simulink model "Simulator_nonlinear_inversion"  (R2015a)
settings: Solver=ode45  StartTime=0.0  StopTime=10  RelTol=1e-3
values from neighbouring files (symbols this model uses):
  A_Servo = [0 1 0; 0 0 1 ; -B0/B3 -B1/B3 -B2/B3]    [Parameters.m]
  b = 0.55/2    (= 0.275)    [Parameters.m]
  B_Servo = [0 ; 0 ; B0/B3]    [Parameters.m]
  C_Servo = eye(3)    [Parameters.m]
  dLMN = [dLdp  0    0 ... (first row only)    [Parameters.m]
  g = 9.81    [Parameters.m]
  I_Pi = diag([8.450e-5 8.450e-5 4.580e-5])    [Parameters.m]
  In = diag([Ixx Iyy Izz])    [Parameters.m]
  InInv = In\eye(3)    [Parameters.m]
  KaD = 5.4    [Parameters.m]
  KaI = 3.6    [Parameters.m]
  KaN = 38    [Parameters.m]
  KaP = 8.0    (= 8)    [Parameters.m]
  Kba = sqrt(KaD/KaI)    [Parameters.m]
  Kbp = sqrt(Kdp/Kip)    [Parameters.m]
  Kbq = sqrt(Kdq/Kiq)    [Parameters.m]
  Kbr = sqrt(Kdr/Kir)    [Parameters.m]
  Kdp = 0.0499    [Parameters.m]
  Kdq = 0.0499    [Parameters.m]
  Kdr = 0.0153    [Parameters.m]
  Kip = 0.304    [Parameters.m]
  Kiq = 0.304    [Parameters.m]
  Kir = 0.125    [Parameters.m]
  KPD = 0.00512    [Parameters.m]
  KPP = 1.61    [Parameters.m]
  Kpp = 0.298    [Parameters.m]
  Kpq = 0.298    [Parameters.m]
  Kpr = 0.135    [Parameters.m]
  Kq = Cq*ro*A*R^3    (= 2.88925724261e-07)    [Parameters.m]
  KRD = 0.00512    [Parameters.m]
  KRP = 1.61    [Parameters.m]
  Kt = Ct*ro*A*R^2    (= 2.46191978476e-05)    [Parameters.m]
  m = 1.510    (= 1.51)    [Parameters.m]
  m_servo = p(1)    [Parameters.m]    (also in model_test_signals.m = 572.9578)
  Mb = diag([m m m])    [Parameters.m]
  MbInv = Mb\eye(3)    [Parameters.m]
  N = 1/Tf    (= 100)    [Parameters.m]
  omega_hover = OMEhov    [Parameters.m]
  pitchMax = pi/6    (= 0.523598775598)    [Parameters.m]
  q_servo = p(2)    [Parameters.m]    (also in model_test_signals.m = 1500)
  rollMax = pi/6    (= 0.523598775598)    [Parameters.m]
  satp = 1.5    [Parameters.m]
  satq = 1.5    [Parameters.m]
  satr = 1    [Parameters.m]
  tau = 0.055257    [Parameters.m]
  U = [-1; 0; 0; 0]    [Main.m]
  x1 = [m q]    [Parameters.m]
  yawRateMax = pi/2    (= 1.57079632679)    [Parameters.m]
undefined symbols (not defined in the file or in its folder): KPI, KRI, sigbuilder_block
libraries: simulink x10, aerolibutil x10
(part 2 of 3)

== system Simulator_nonlinear_inversion/TiltCopter/Actuators/External Momentum_2 ==
  tau_pi : Inport
  alpha_i : Inport  Port=2
  omega_i : Inport  Port=3
  motor_number : Inport  Port=4
  3x3 Cross Product : aerolibutil/3x3 Cross Product
  O_BPi : MATLAB Function  TreatAsAtomicUnit=on
  Product : Product  Multiplication=Matrix(*)
  Product1 : Product  Multiplication=Matrix(*)
  R_BP2 : MATLAB Function  TreatAsAtomicUnit=on
  Sum : Sum  Inputs=-+|
  Thrust computation : Subsystem
  M_i : Outport
  wires:
  Sum/1 -> M_i/1
  R_BP2/1(Rotation_matrix) -> Product1/1, Product/1
  alpha_i/1 -> R_BP2/1(alpha_2)
  Product/1 -> 3x3 Cross Product/2
  tau_pi/1 -> Product1/2
  motor_number/1 -> O_BPi/1(motor_number)
  omega_i/1 -> Thrust computation/1(omega_i)
  Thrust computation/1(Vector_Thrust_i) -> Product/2
  3x3 Cross Product/1 -> Sum/2
  Product1/1 -> Sum/1
  O_BPi/1(Origin_Rotation) -> 3x3 Cross Product/1

== system Simulator_nonlinear_inversion/TiltCopter/Actuators/External Momentum_3 ==
  tau_pi : Inport
  alpha_i : Inport  Port=2
  omega_i : Inport  Port=3
  motor_number : Inport  Port=4
  3x3 Cross Product : aerolibutil/3x3 Cross Product
  O_BPi : MATLAB Function  TreatAsAtomicUnit=on
  Product : Product  Multiplication=Matrix(*)
  Product1 : Product  Multiplication=Matrix(*)
  R_BP3 : MATLAB Function  TreatAsAtomicUnit=on
  Sum : Sum  Inputs=-+|
  Thrust computation : Subsystem
  M_i : Outport
  wires:
  Sum/1 -> M_i/1
  R_BP3/1(Rotation_matrix) -> Product1/1, Product/1
  alpha_i/1 -> R_BP3/1(alpha_3)
  Product/1 -> 3x3 Cross Product/2
  tau_pi/1 -> Product1/2
  motor_number/1 -> O_BPi/1(motor_number)
  omega_i/1 -> Thrust computation/1(omega_i)
  Thrust computation/1(Vector_Thrust_i) -> Product/2
  3x3 Cross Product/1 -> Sum/2
  Product1/1 -> Sum/1
  O_BPi/1(Origin_Rotation) -> 3x3 Cross Product/1

== system Simulator_nonlinear_inversion/TiltCopter/Actuators/External Momentum_4 ==
  tau_pi : Inport
  alpha_i : Inport  Port=2
  omega_i : Inport  Port=3
  motor_number : Inport  Port=4
  3x3 Cross Product : aerolibutil/3x3 Cross Product
  O_BPi : MATLAB Function  TreatAsAtomicUnit=on
  Product : Product  Multiplication=Matrix(*)
  Product1 : Product  Multiplication=Matrix(*)
  R_BP4 : MATLAB Function  TreatAsAtomicUnit=on
  Sum : Sum  Inputs=-+|
  Thrust computation : Subsystem
  M_i : Outport
  wires:
  Sum/1 -> M_i/1
  R_BP4/1(Rotation_matrix) -> Product1/1, Product/1
  alpha_i/1 -> R_BP4/1(alpha_4)
  Product/1 -> 3x3 Cross Product/2
  tau_pi/1 -> Product1/2
  motor_number/1 -> O_BPi/1(motor_number)
  omega_i/1 -> Thrust computation/1(omega_i)
  Thrust computation/1(Vector_Thrust_i) -> Product/2
  3x3 Cross Product/1 -> Sum/2
  Product1/1 -> Sum/1
  O_BPi/1(Origin_Rotation) -> 3x3 Cross Product/1

== system Simulator_nonlinear_inversion/TiltCopter/Actuators/Servo_Motor 1 ==
  Alpha_1 [deg] : Inport
  Demux : Demux  Outputs=3
  State-Space : StateSpace  A=A_Servo  B=B_Servo  C=C_Servo  D=[0 0 0]'  X0=[0 0 0 ]  ContinuousStateAttributes=['alpha' 'dalpha' 'ddalpha']
  deg2rad : Gain  Gain=pi/180
  alpha_1 [rad] : Outport
  dalpha_1 : Outport  Port=2
  ddalpha_1 : Outport  Port=3
  wires:
  deg2rad/1 -> State-Space/1
  Alpha_1 [deg]/1 -> deg2rad/1
  State-Space/1 -> Demux/1
  Demux/1 -> alpha_1 [rad]/1
  Demux/2 -> dalpha_1/1
  Demux/3 -> ddalpha_1/1

== system Simulator_nonlinear_inversion/TiltCopter/Actuators/Servo_Motor 2 ==
  Alpha_2 [deg] : Inport
  Demux : Demux  Outputs=3
  State-Space : StateSpace  A=A_Servo  B=B_Servo  C=C_Servo  D=[0 0 0]'  X0=[0 0 0 ]  ContinuousStateAttributes=['alpha' 'dalpha' 'ddalpha']
  deg2rad : Gain  Gain=pi/180
  alpha_2 [rad] : Outport
  dalpha_2 : Outport  Port=2
  ddalpha_2 : Outport  Port=3
  wires:
  State-Space/1 -> Demux/1
  Demux/3 -> ddalpha_2/1
  Demux/2 -> dalpha_2/1
  Demux/1 -> alpha_2 [rad]/1
  deg2rad/1 -> State-Space/1
  Alpha_2 [deg]/1 -> deg2rad/1

== system Simulator_nonlinear_inversion/TiltCopter/Actuators/Servo_Motor 3 ==
  Alpha_3 [deg] : Inport
  Demux : Demux  Outputs=3
  State-Space : StateSpace  A=A_Servo  B=B_Servo  C=C_Servo  D=[0 0 0]'  X0=[0 0 0 ]  ContinuousStateAttributes=['alpha' 'dalpha' 'ddalpha']
  deg2rad : Gain  Gain=pi/180
  alpha_3 [rad] : Outport
  dalpha_3 : Outport  Port=2
  ddalpha_3 : Outport  Port=3
  wires:
  Demux/1 -> alpha_3 [rad]/1
  Demux/2 -> dalpha_3/1
  Demux/3 -> ddalpha_3/1
  deg2rad/1 -> State-Space/1
  Alpha_3 [deg]/1 -> deg2rad/1
  State-Space/1 -> Demux/1

== system Simulator_nonlinear_inversion/TiltCopter/Actuators/Servo_Motor 4 ==
  Alpha_4 [deg] : Inport
  Demux : Demux  Outputs=3
  State-Space : StateSpace  A=A_Servo  B=B_Servo  C=C_Servo  D=[0 0 0]'  X0=[0 0 0 ]  ContinuousStateAttributes=['alpha' 'dalpha' 'ddalpha']
  deg2rad : Gain  Gain=pi/180
  alpha_4 [rad] : Outport
  dalpha_4 : Outport  Port=2
  ddalpha_4 : Outport  Port=3
  wires:
  Demux/1 -> alpha_4 [rad]/1
  Demux/2 -> dalpha_4/1
  Demux/3 -> ddalpha_4/1
  deg2rad/1 -> State-Space/1
  Alpha_4 [deg]/1 -> deg2rad/1
  State-Space/1 -> Demux/1

== system Simulator_nonlinear_inversion/TiltCopter/Actuators/Traslational Force_1 ==
  alpha_i : Inport
  omega_i : Inport  Port=2
  Product : Product  Multiplication=Matrix(*)
  R_BP1 : MATLAB Function  TreatAsAtomicUnit=on
  Thrust computation : Subsystem
  F_i : Outport
  wires:
  Thrust computation/1(Vector_Thrust_i) -> Product/2
  Product/1 -> F_i/1
  omega_i/1 -> Thrust computation/1(omega_i)
  R_BP1/1(Rotation_matrix) -> Product/1
  alpha_i/1 -> R_BP1/1(alpha_1)

== system Simulator_nonlinear_inversion/TiltCopter/Actuators/Traslational Force_2 ==
  alpha_i : Inport
  omega_i : Inport  Port=2
  Product : Product  Multiplication=Matrix(*)
  R_BP2 : MATLAB Function  TreatAsAtomicUnit=on
  Thrust computation : Subsystem
  F_i : Outport
  wires:
  Thrust computation/1(Vector_Thrust_i) -> Product/2
  Product/1 -> F_i/1
  omega_i/1 -> Thrust computation/1(omega_i)
  R_BP2/1(Rotation_matrix) -> Product/1
  alpha_i/1 -> R_BP2/1(alpha_2)

== system Simulator_nonlinear_inversion/TiltCopter/Actuators/Traslational Force_3 ==
  alpha_i : Inport
  omega_i : Inport  Port=2
  Product : Product  Multiplication=Matrix(*)
  R_BP3 : MATLAB Function  TreatAsAtomicUnit=on
  Thrust computation : Subsystem
  F_i : Outport
  wires:
  Thrust computation/1(Vector_Thrust_i) -> Product/2
  Product/1 -> F_i/1
  omega_i/1 -> Thrust computation/1(omega_i)
  R_BP3/1(Rotation_matrix) -> Product/1
  alpha_i/1 -> R_BP3/1(alpha_3)

== system Simulator_nonlinear_inversion/TiltCopter/Actuators/Traslational Force_4 ==
  alpha_i : Inport
  omega_i : Inport  Port=2
  Product : Product  Multiplication=Matrix(*)
  R_BP4 : MATLAB Function  TreatAsAtomicUnit=on
  Thrust computation : Subsystem
  F_i : Outport
  wires:
  Thrust computation/1(Vector_Thrust_i) -> Product/2
  Product/1 -> F_i/1
  omega_i/1 -> Thrust computation/1(omega_i)
  R_BP4/1(Rotation_matrix) -> Product/1
  alpha_i/1 -> R_BP4/1(alpha_4)

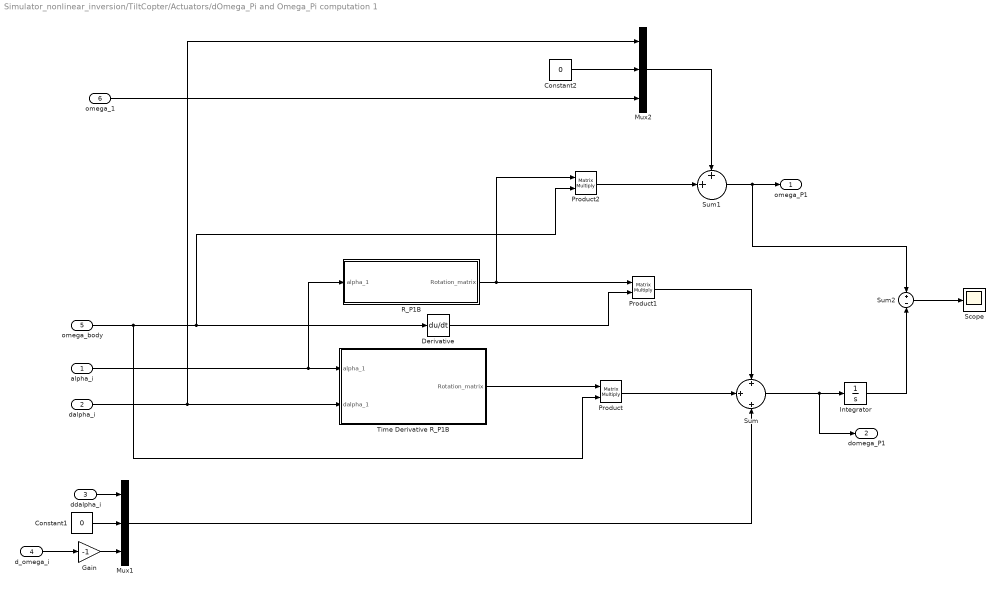
== system Simulator_nonlinear_inversion/TiltCopter/Actuators/dOmega_Pi and Omega_Pi computation 1 ==
  alpha_i : Inport
  dalpha_i : Inport  Port=2
  ddalpha_i : Inport  Port=3
  d_omega_i : Inport  Port=4
  omega_body : Inport  Port=5
  omega_1 : Inport  Port=6
  Constant1 : Constant  Value=0
  Constant2 : Constant  Value=0
  Derivative : Derivative
  Gain : Gain  Gain=-1
  Integrator : Integrator
  Mux1 : Mux  Inputs=3
  Mux2 : Mux  Inputs=3
  Product : Product  Multiplication=Matrix(*)
  Product1 : Product  Multiplication=Matrix(*)
  Product2 : Product  Multiplication=Matrix(*)
  R_P1B : MATLAB Function  TreatAsAtomicUnit=on
  Scope : Scope
      settings: ShowLegends=on  YMin=-10  YMax=10  SaveName=ScopeData29
  Sum : Sum  Inputs=+|+|+
  Sum1 : Sum  Inputs=++|
  Sum2 : Sum  Inputs=+-
  Time Derivative R_P1B : MATLAB Function  TreatAsAtomicUnit=on
  omega_P1 : Outport
  domega_P1 : Outport  Port=2
  wires:
  Derivative/1 -> Product1/2
  Product/1 -> Sum/2
  Time Derivative R_P1B/1(Rotation_matrix) -> Product/1
  Constant1/1 -> Mux1/2
  omega_body/1 -> Product/2, Product2/2, Derivative/1
  dalpha_i/1 -> Mux2/1, Time Derivative R_P1B/2(dalpha_1)
  alpha_i/1 -> R_P1B/1(alpha_1), Time Derivative R_P1B/1(alpha_1)
  R_P1B/1(Rotation_matrix) -> Product2/1, Product1/1
  Sum/1 -> domega_P1/1, Integrator/1
  Product1/1 -> Sum/1
  Mux1/1 -> Sum/3
  ddalpha_i/1 -> Mux1/1
  Product2/1 -> Sum1/2
  Constant2/1 -> Mux2/2
  Mux2/1 -> Sum1/1
  Sum1/1 -> Sum2/1, omega_P1/1
  omega_1/1 -> Mux2/3
  d_omega_i/1 -> Gain/1
  Integrator/1 -> Sum2/2
  Sum2/1 -> Scope/1
  Gain/1 -> Mux1/3

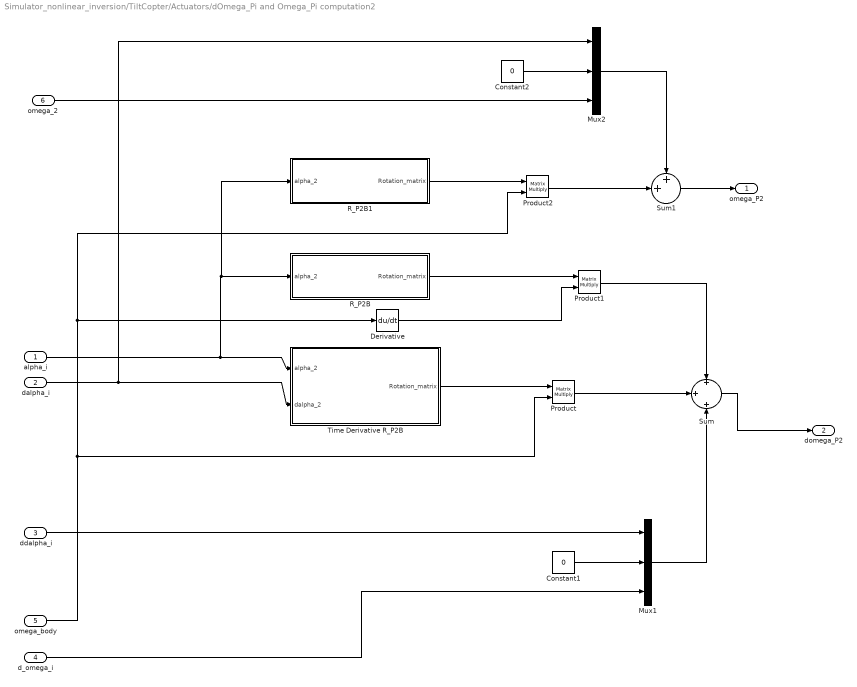
== system Simulator_nonlinear_inversion/TiltCopter/Actuators/dOmega_Pi and Omega_Pi computation2 ==
  alpha_i : Inport
  dalpha_i : Inport  Port=2
  ddalpha_i : Inport  Port=3
  d_omega_i : Inport  Port=4
  omega_body : Inport  Port=5
  omega_2 : Inport  Port=6
  Constant1 : Constant  Value=0
  Constant2 : Constant  Value=0
  Derivative : Derivative
  Mux1 : Mux  Inputs=3
  Mux2 : Mux  Inputs=3
  Product : Product  Multiplication=Matrix(*)
  Product1 : Product  Multiplication=Matrix(*)
  Product2 : Product  Multiplication=Matrix(*)
  R_P2B : MATLAB Function  TreatAsAtomicUnit=on
  R_P2B1 : MATLAB Function  TreatAsAtomicUnit=on
  Sum : Sum  Inputs=+|+|+
  Sum1 : Sum  Inputs=++|
  Time Derivative R_P2B : MATLAB Function  TreatAsAtomicUnit=on
  omega_P2 : Outport
  domega_P2 : Outport  Port=2
  wires:
  Derivative/1 -> Product1/2
  Product/1 -> Sum/2
  Time Derivative R_P2B/1(Rotation_matrix) -> Product/1
  Constant1/1 -> Mux1/2
  omega_body/1 -> Product/2, Product2/2, Derivative/1
  dalpha_i/1 -> Mux2/1, Time Derivative R_P2B/2(dalpha_2)
  alpha_i/1 -> R_P2B1/1(alpha_2), R_P2B/1(alpha_2), Time Derivative R_P2B/1(alpha_2)
  Sum/1 -> domega_P2/1
  Product1/1 -> Sum/1
  Mux1/1 -> Sum/3
  ddalpha_i/1 -> Mux1/1
  R_P2B/1(Rotation_matrix) -> Product1/1
  R_P2B1/1(Rotation_matrix) -> Product2/1
  Product2/1 -> Sum1/2
  Constant2/1 -> Mux2/2
  Mux2/1 -> Sum1/1
  Sum1/1 -> omega_P2/1
  d_omega_i/1 -> Mux1/3
  omega_2/1 -> Mux2/3

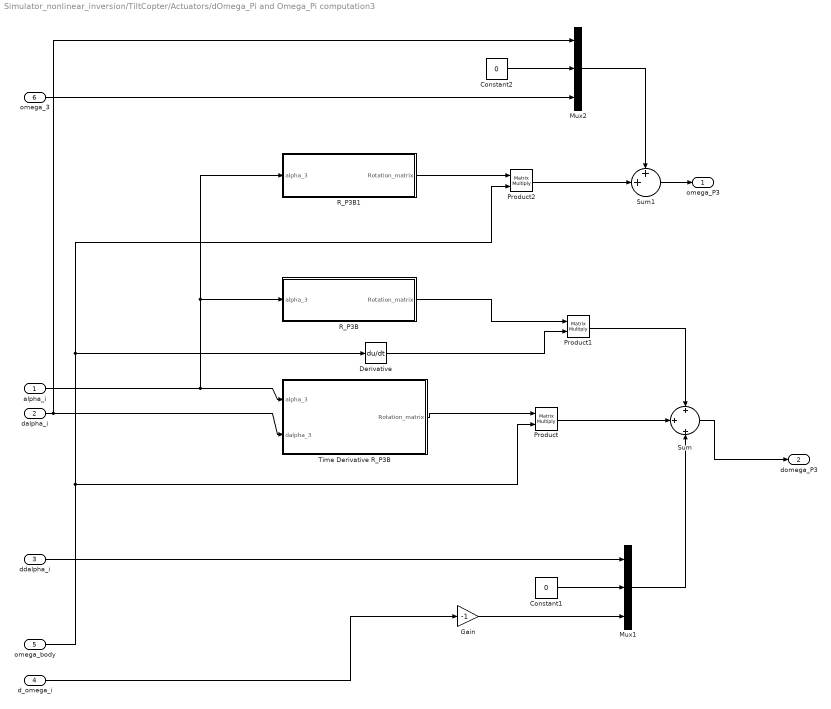
== system Simulator_nonlinear_inversion/TiltCopter/Actuators/dOmega_Pi and Omega_Pi computation3 ==
  alpha_i : Inport
  dalpha_i : Inport  Port=2
  ddalpha_i : Inport  Port=3
  d_omega_i : Inport  Port=4
  omega_body : Inport  Port=5
  omega_3 : Inport  Port=6
  Constant1 : Constant  Value=0
  Constant2 : Constant  Value=0
  Derivative : Derivative
  Gain : Gain  Gain=-1
  Mux1 : Mux  Inputs=3
  Mux2 : Mux  Inputs=3
  Product : Product  Multiplication=Matrix(*)
  Product1 : Product  Multiplication=Matrix(*)
  Product2 : Product  Multiplication=Matrix(*)
  R_P3B : MATLAB Function  TreatAsAtomicUnit=on
  R_P3B1 : MATLAB Function  TreatAsAtomicUnit=on
  Sum : Sum  Inputs=+|+|+
  Sum1 : Sum  Inputs=++|
  Time Derivative R_P3B : MATLAB Function  TreatAsAtomicUnit=on
  omega_P3 : Outport
  domega_P3 : Outport  Port=2
  wires:
  Derivative/1 -> Product1/2
  Product/1 -> Sum/2
  Time Derivative R_P3B/1(Rotation_matrix) -> Product/1
  Constant1/1 -> Mux1/2
  omega_body/1 -> Product/2, Product2/2, Derivative/1
  alpha_i/1 -> R_P3B1/1(alpha_3), R_P3B/1(alpha_3), Time Derivative R_P3B/1(alpha_3)
  Sum/1 -> domega_P3/1
  Product1/1 -> Sum/1
  Mux1/1 -> Sum/3
  ddalpha_i/1 -> Mux1/1
  R_P3B/1(Rotation_matrix) -> Product1/1
  R_P3B1/1(Rotation_matrix) -> Product2/1
  Product2/1 -> Sum1/2
  Constant2/1 -> Mux2/2
  Mux2/1 -> Sum1/1
  dalpha_i/1 -> Mux2/1, Time Derivative R_P3B/2(dalpha_3)
  Sum1/1 -> omega_P3/1
  d_omega_i/1 -> Gain/1
  omega_3/1 -> Mux2/3
  Gain/1 -> Mux1/3

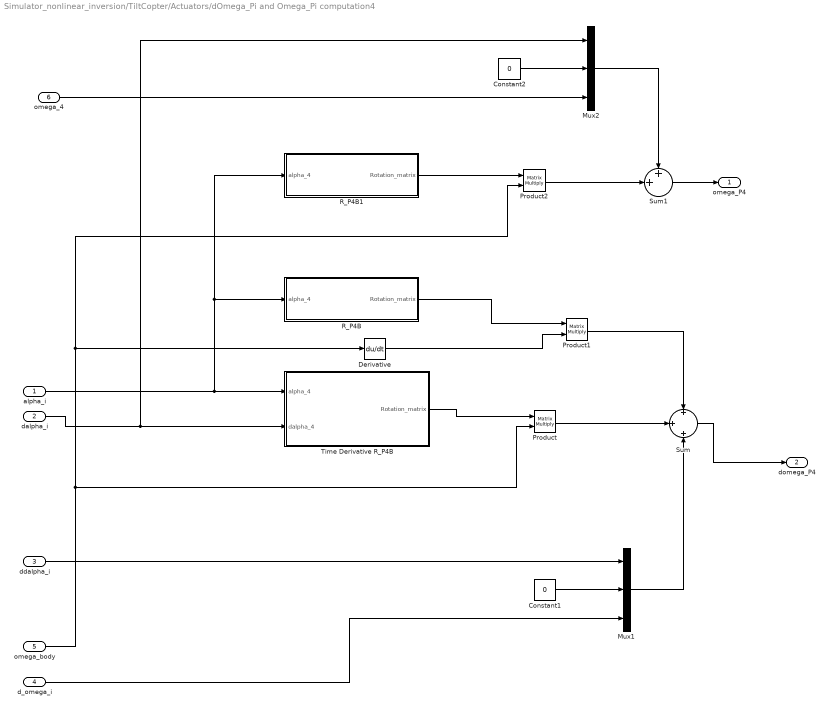
== system Simulator_nonlinear_inversion/TiltCopter/Actuators/dOmega_Pi and Omega_Pi computation4 ==
  alpha_i : Inport
  dalpha_i : Inport  Port=2
  ddalpha_i : Inport  Port=3
  d_omega_i : Inport  Port=4
  omega_body : Inport  Port=5
  omega_4 : Inport  Port=6
  Constant1 : Constant  Value=0
  Constant2 : Constant  Value=0
  Derivative : Derivative
  Mux1 : Mux  Inputs=3
  Mux2 : Mux  Inputs=3
  Product : Product  Multiplication=Matrix(*)
  Product1 : Product  Multiplication=Matrix(*)
  Product2 : Product  Multiplication=Matrix(*)
  R_P4B : MATLAB Function  TreatAsAtomicUnit=on
  R_P4B1 : MATLAB Function  TreatAsAtomicUnit=on
  Sum : Sum  Inputs=+|+|+
  Sum1 : Sum  Inputs=++|
  Time Derivative R_P4B : MATLAB Function  TreatAsAtomicUnit=on
  omega_P4 : Outport
  domega_P4 : Outport  Port=2
  wires:
  Derivative/1 -> Product1/2
  Product/1 -> Sum/2
  Time Derivative R_P4B/1(Rotation_matrix) -> Product/1
  Constant1/1 -> Mux1/2
  omega_body/1 -> Product/2, Product2/2, Derivative/1
  dalpha_i/1 -> Mux2/1, Time Derivative R_P4B/2(dalpha_4)
  alpha_i/1 -> R_P4B1/1(alpha_4), R_P4B/1(alpha_4), Time Derivative R_P4B/1(alpha_4)
  Sum/1 -> domega_P4/1
  Product1/1 -> Sum/1
  Mux1/1 -> Sum/3
  ddalpha_i/1 -> Mux1/1
  R_P4B/1(Rotation_matrix) -> Product1/1
  Product2/1 -> Sum1/2
  Constant2/1 -> Mux2/2
  Mux2/1 -> Sum1/1
  R_P4B1/1(Rotation_matrix) -> Product2/1
  Sum1/1 -> omega_P4/1
  omega_4/1 -> Mux2/3
  d_omega_i/1 -> Mux1/3

== system Simulator_nonlinear_inversion/TiltCopter/Actuators/tau_p1 computation ==
  omega_P1 : Inport
  domega_P1 : Inport  Port=2
  omega_i : Inport  Port=3
  3x3 Cross Product : aerolibutil/3x3 Cross Product
  Constant : Constant  Value=I_Pi
  Drag torque computation : Subsystem
  Gain : Gain  Gain=[1;1;-1]
  Product : Product  Multiplication=Matrix(*)
  Product1 : Product  Multiplication=Matrix(*)
  Sum : Sum  Inputs=+|+|-
  tau_P1 : Outport
  wires:
  Constant/1 -> Product/1, Product1/1
  omega_P1/1 -> 3x3 Cross Product/1, Product1/2
  Product/1 -> Sum/2
  domega_P1/1 -> Product/2
  Product1/1 -> 3x3 Cross Product/2
  Sum/1 -> tau_P1/1
  3x3 Cross Product/1 -> Sum/1
  Drag torque computation/1(Vector_DragTorque_i) -> Gain/1
  omega_i/1 -> Drag torque computation/1(omega_P1_z)
  Gain/1 -> Sum/3

== system Simulator_nonlinear_inversion/TiltCopter/Actuators/tau_p2 computation ==
  omega_P2 : Inport
  domega_P2 : Inport  Port=2
  omega_i : Inport  Port=3
  3x3 Cross Product : aerolibutil/3x3 Cross Product
  Constant : Constant  Value=I_Pi
  Drag torque computation : Subsystem
  Gain : Gain  Gain=[1;1;-1]
  Product : Product  Multiplication=Matrix(*)
  Product1 : Product  Multiplication=Matrix(*)
  Sum : Sum  Inputs=+|+|-
  tau_P2 : Outport
  wires:
  3x3 Cross Product/1 -> Sum/1
  Sum/1 -> tau_P2/1
  Product1/1 -> 3x3 Cross Product/2
  domega_P2/1 -> Product/2
  Product/1 -> Sum/2
  omega_P2/1 -> Product1/2, 3x3 Cross Product/1
  Constant/1 -> Product/1, Product1/1
  Drag torque computation/1(Vector_DragTorque_i) -> Gain/1
  omega_i/1 -> Drag torque computation/1(omega_P2)
  Gain/1 -> Sum/3

== system Simulator_nonlinear_inversion/TiltCopter/Actuators/tau_p3 computation1 ==
  omega_P3 : Inport
  domega_P3 : Inport  Port=2
  omega_i : Inport  Port=3
  3x3 Cross Product : aerolibutil/3x3 Cross Product
  Constant : Constant  Value=I_Pi
  Drag torque computation : Subsystem
  Gain : Gain  Gain=[1;1;-1]
  Product : Product  Multiplication=Matrix(*)
  Product1 : Product  Multiplication=Matrix(*)
  Sum : Sum  Inputs=+|+|-
  tau_P3 : Outport
  wires:
  Constant/1 -> Product1/1, Product/1
  omega_P3/1 -> 3x3 Cross Product/1, Product1/2
  Product/1 -> Sum/2
  domega_P3/1 -> Product/2
  Product1/1 -> 3x3 Cross Product/2
  Sum/1 -> tau_P3/1
  3x3 Cross Product/1 -> Sum/1
  Drag torque computation/1(Vector_DragTorque_i) -> Gain/1
  omega_i/1 -> Drag torque computation/1(omega_P3)
  Gain/1 -> Sum/3

== system Simulator_nonlinear_inversion/TiltCopter/Actuators/tau_p4 computation2 ==
  omega_P4 : Inport
  domega_P4 : Inport  Port=2
  omega_i : Inport  Port=3
  3x3 Cross Product : aerolibutil/3x3 Cross Product
  Constant : Constant  Value=I_Pi
  Drag torque computation : Subsystem
  Gain : Gain  Gain=[1;1;-1]
  Product : Product  Multiplication=Matrix(*)
  Product1 : Product  Multiplication=Matrix(*)
  Sum : Sum  Inputs=+|+|-
  tau_P4 : Outport
  wires:
  3x3 Cross Product/1 -> Sum/1
  Sum/1 -> tau_P4/1
  Product1/1 -> 3x3 Cross Product/2
  domega_P4/1 -> Product/2
  Product/1 -> Sum/2
  omega_P4/1 -> Product1/2, 3x3 Cross Product/1
  Constant/1 -> Product/1, Product1/1
  Drag torque computation/1(Vector_DragTorque_i) -> Gain/1
  omega_i/1 -> Drag torque computation/1(omega_P4)
  Gain/1 -> Sum/3

== system Simulator_nonlinear_inversion/TiltCopter/Actuators/ESC+Brushless1/Subsystem ==
  Throttle [%] : Inport
  Bias : Bias  Bias=x1(2)
  Gain : Gain  Gain=x1(1)
  Gain1 : Gain  Gain=-1/tau
  Gain2 : Gain  Gain=1/tau
  Gain3 : Gain  Gain=x1(1)
  Gain4 : Gain  Gain=x1(1)
  Sum : Sum  Inputs=|++
  Transfer Fcn : TransferFcn  Denominator=[(tau) 1]
  Transfer Fcn1 : TransferFcn  Denominator=[(tau) 1]
  omega_i : Outport
  domega_i : Outport  Port=2
  wires:
  Throttle [%]/1 -> Gain4/1, Transfer Fcn1/1, Transfer Fcn/1
  Transfer Fcn1/1 -> Gain1/1
  Gain1/1 -> Gain3/1
  Sum/1 -> domega_i/1
  Gain2/1 -> Sum/2
  Gain3/1 -> Sum/1
  Bias/1 -> omega_i/1
  Gain/1 -> Bias/1
  Transfer Fcn/1 -> Gain/1
  Gain4/1 -> Gain2/1

== system Simulator_nonlinear_inversion/TiltCopter/Actuators/ESC+Brushless2/Subsystem ==
  Throttle [%] : Inport
  Bias : Bias  Bias=x1(2)
  Gain : Gain  Gain=x1(1)
  Gain1 : Gain  Gain=-1/tau
  Gain2 : Gain  Gain=1/tau
  Gain3 : Gain  Gain=x1(1)
  Gain4 : Gain  Gain=x1(1)
  Sum : Sum  Inputs=|++
  Transfer Fcn : TransferFcn  Denominator=[(tau) 1]
  Transfer Fcn1 : TransferFcn  Denominator=[(tau) 1]
  omega_i : Outport
  domega_i : Outport  Port=2
  wires:
  Throttle [%]/1 -> Gain4/1, Transfer Fcn1/1, Transfer Fcn/1
  Transfer Fcn1/1 -> Gain1/1
  Gain1/1 -> Gain3/1
  Sum/1 -> domega_i/1
  Gain2/1 -> Sum/2
  Gain3/1 -> Sum/1
  Bias/1 -> omega_i/1
  Gain/1 -> Bias/1
  Transfer Fcn/1 -> Gain/1
  Gain4/1 -> Gain2/1

== system Simulator_nonlinear_inversion/TiltCopter/Actuators/ESC+Brushless3/Subsystem ==
  Throttle [%] : Inport
  Bias : Bias  Bias=x1(2)
  Gain : Gain  Gain=x1(1)
  Gain1 : Gain  Gain=-1/tau
  Gain2 : Gain  Gain=1/tau
  Gain3 : Gain  Gain=x1(1)
  Gain4 : Gain  Gain=x1(1)
  Sum : Sum  Inputs=|++
  Transfer Fcn : TransferFcn  Denominator=[(tau) 1]
  Transfer Fcn1 : TransferFcn  Denominator=[(tau) 1]
  omega_i : Outport
  domega_i : Outport  Port=2
  wires:
  Throttle [%]/1 -> Gain4/1, Transfer Fcn1/1, Transfer Fcn/1
  Transfer Fcn1/1 -> Gain1/1
  Gain1/1 -> Gain3/1
  Sum/1 -> domega_i/1
  Gain2/1 -> Sum/2
  Gain3/1 -> Sum/1
  Bias/1 -> omega_i/1
  Gain/1 -> Bias/1
  Transfer Fcn/1 -> Gain/1
  Gain4/1 -> Gain2/1

== system Simulator_nonlinear_inversion/TiltCopter/Actuators/ESC+Brushless4/Subsystem ==
  Throttle [%] : Inport
  Bias : Bias  Bias=x1(2)
  Gain : Gain  Gain=x1(1)
  Gain1 : Gain  Gain=-1/tau
  Gain2 : Gain  Gain=1/tau
  Gain3 : Gain  Gain=x1(1)
  Gain4 : Gain  Gain=x1(1)
  Sum : Sum  Inputs=|++
  Transfer Fcn : TransferFcn  Denominator=[(tau) 1]
  Transfer Fcn1 : TransferFcn  Denominator=[(tau) 1]
  omega_i : Outport
  domega_i : Outport  Port=2
  wires:
  Throttle [%]/1 -> Gain4/1, Transfer Fcn1/1, Transfer Fcn/1
  Transfer Fcn1/1 -> Gain1/1
  Gain1/1 -> Gain3/1
  Sum/1 -> domega_i/1
  Gain2/1 -> Sum/2
  Gain3/1 -> Sum/1
  Bias/1 -> omega_i/1
  Gain/1 -> Bias/1
  Transfer Fcn/1 -> Gain/1
  Gain4/1 -> Gain2/1

== system Simulator_nonlinear_inversion/TiltCopter/Actuators/External Momentum_1/Thrust computation ==
  omega_i : Inport
  Constant : Constant  Value=-Kt
  Constant1 : Constant  Value=0
  Constant2 : Constant  Value=0
  Mux : Mux  Inputs=3
  Product : Product
  Product1 : Product
  Vector_Thrust_i : Outport
  wires:
  Constant2/1 -> Mux/2
  omega_i/1 -> Product/2, Product/1
  Product/1 -> Product1/1
  Constant1/1 -> Mux/1
  Mux/1 -> Vector_Thrust_i/1
  Product1/1 -> Mux/3
  Constant/1 -> Product1/2

== system Simulator_nonlinear_inversion/TiltCopter/Actuators/External Momentum_2/Thrust computation ==
  omega_i : Inport
  Constant : Constant  Value=-Kt
  Constant1 : Constant  Value=0
  Constant2 : Constant  Value=0
  Mux : Mux  Inputs=3
  Product : Product
  Product1 : Product
  Vector_Thrust_i : Outport
  wires:
  Constant2/1 -> Mux/2
  omega_i/1 -> Product/2, Product/1
  Product/1 -> Product1/1
  Constant1/1 -> Mux/1
  Mux/1 -> Vector_Thrust_i/1
  Product1/1 -> Mux/3
  Constant/1 -> Product1/2

== system Simulator_nonlinear_inversion/TiltCopter/Actuators/External Momentum_3/Thrust computation ==
  omega_i : Inport
  Constant : Constant  Value=-Kt
  Constant1 : Constant  Value=0
  Constant2 : Constant  Value=0
  Mux : Mux  Inputs=3
  Product : Product
  Product1 : Product
  Vector_Thrust_i : Outport
  wires:
  Constant2/1 -> Mux/2
  omega_i/1 -> Product/2, Product/1
  Product/1 -> Product1/1
  Constant1/1 -> Mux/1
  Mux/1 -> Vector_Thrust_i/1
  Product1/1 -> Mux/3
  Constant/1 -> Product1/2

== system Simulator_nonlinear_inversion/TiltCopter/Actuators/External Momentum_4/Thrust computation ==
  omega_i : Inport
  Constant : Constant  Value=-Kt
  Constant1 : Constant  Value=0
  Constant2 : Constant  Value=0
  Mux : Mux  Inputs=3
  Product : Product
  Product1 : Product
  Vector_Thrust_i : Outport
  wires:
  Constant2/1 -> Mux/2
  omega_i/1 -> Product/2, Product/1
  Product/1 -> Product1/1
  Constant1/1 -> Mux/1
  Mux/1 -> Vector_Thrust_i/1
  Product1/1 -> Mux/3
  Constant/1 -> Product1/2

== system Simulator_nonlinear_inversion/TiltCopter/Actuators/Traslational Force_1/Thrust computation ==
  omega_i : Inport
  Constant : Constant  Value=-Kt
  Constant1 : Constant  Value=0
  Constant2 : Constant  Value=0
  Mux : Mux  Inputs=3
  Product : Product
  Product1 : Product
  Vector_Thrust_i : Outport
  wires:
  Constant2/1 -> Mux/2
  omega_i/1 -> Product/2, Product/1
  Product/1 -> Product1/1
  Constant1/1 -> Mux/1
  Mux/1 -> Vector_Thrust_i/1
  Product1/1 -> Mux/3
  Constant/1 -> Product1/2

== system Simulator_nonlinear_inversion/TiltCopter/Actuators/Traslational Force_2/Thrust computation ==
  omega_i : Inport
  Constant : Constant  Value=-Kt
  Constant1 : Constant  Value=0
  Constant2 : Constant  Value=0
  Mux : Mux  Inputs=3
  Product : Product
  Product1 : Product
  Vector_Thrust_i : Outport
  wires:
  Constant2/1 -> Mux/2
  omega_i/1 -> Product/2, Product/1
  Product/1 -> Product1/1
  Constant1/1 -> Mux/1
  Mux/1 -> Vector_Thrust_i/1
  Product1/1 -> Mux/3
  Constant/1 -> Product1/2

== system Simulator_nonlinear_inversion/TiltCopter/Actuators/Traslational Force_3/Thrust computation ==
  omega_i : Inport
  Constant : Constant  Value=-Kt
  Constant1 : Constant  Value=0
  Constant2 : Constant  Value=0
  Mux : Mux  Inputs=3
  Product : Product
  Product1 : Product
  Vector_Thrust_i : Outport
  wires:
  Constant2/1 -> Mux/2
  omega_i/1 -> Product/2, Product/1
  Product/1 -> Product1/1
  Constant1/1 -> Mux/1
  Mux/1 -> Vector_Thrust_i/1
  Product1/1 -> Mux/3
  Constant/1 -> Product1/2

== system Simulator_nonlinear_inversion/TiltCopter/Actuators/Traslational Force_4/Thrust computation ==
  omega_i : Inport
  Constant : Constant  Value=-Kt
  Constant1 : Constant  Value=0
  Constant2 : Constant  Value=0
  Mux : Mux  Inputs=3
  Product : Product
  Product1 : Product
  Vector_Thrust_i : Outport
  wires:
  Constant2/1 -> Mux/2
  omega_i/1 -> Product/2, Product/1
  Product/1 -> Product1/1
  Constant1/1 -> Mux/1
  Mux/1 -> Vector_Thrust_i/1
  Product1/1 -> Mux/3
  Constant/1 -> Product1/2

== system Simulator_nonlinear_inversion/TiltCopter/Actuators/tau_p1 computation/Drag torque computation ==
  omega_P1_z : Inport
  Constant : Constant  Value=-Kq
  Constant1 : Constant  Value=0
  Constant2 : Constant  Value=0
  Mux : Mux  Inputs=3
  Product : Product
  Product1 : Product
  Vector_DragTorque_i : Outport
  wires:
  Constant2/1 -> Mux/2
  Product/1 -> Product1/1
  Constant1/1 -> Mux/1
  Mux/1 -> Vector_DragTorque_i/1
  Product1/1 -> Mux/3
  Constant/1 -> Product1/2
  omega_P1_z/1 -> Product/2, Product/1

== system Simulator_nonlinear_inversion/TiltCopter/Actuators/tau_p2 computation/Drag torque computation ==
  omega_P2 : Inport
  Constant : Constant  Value=Kq
  Constant1 : Constant  Value=0
  Constant2 : Constant  Value=0
  Mux : Mux  Inputs=3
  Product : Product
  Product1 : Product
  Vector_DragTorque_i : Outport
  wires:
  Constant2/1 -> Mux/2
  Product/1 -> Product1/1
  Constant1/1 -> Mux/1
  Mux/1 -> Vector_DragTorque_i/1
  Product1/1 -> Mux/3
  Constant/1 -> Product1/2
  omega_P2/1 -> Product/2, Product/1

== system Simulator_nonlinear_inversion/TiltCopter/Actuators/tau_p3 computation1/Drag torque computation ==
  omega_P3 : Inport
  Constant : Constant  Value=-Kq
  Constant1 : Constant  Value=0
  Constant2 : Constant  Value=0
  Mux : Mux  Inputs=3
  Product : Product
  Product1 : Product
  Vector_DragTorque_i : Outport
  wires:
  Constant2/1 -> Mux/2
  Product/1 -> Product1/1
  Constant1/1 -> Mux/1
  Mux/1 -> Vector_DragTorque_i/1
  Product1/1 -> Mux/3
  Constant/1 -> Product1/2
  omega_P3/1 -> Product/2, Product/1

== system Simulator_nonlinear_inversion/TiltCopter/Actuators/tau_p4 computation2/Drag torque computation ==
  omega_P4 : Inport
  Constant : Constant  Value=Kq
  Constant1 : Constant  Value=0
  Constant2 : Constant  Value=0
  Mux : Mux  Inputs=3
  Product : Product
  Product1 : Product
  Vector_DragTorque_i : Outport
  wires:
  Constant2/1 -> Mux/2
  Product/1 -> Product1/1
  Constant1/1 -> Mux/1
  Mux/1 -> Vector_DragTorque_i/1
  Product1/1 -> Mux/3
  Constant/1 -> Product1/2
  omega_P4/1 -> Product/2, Product/1

== matlab function Simulator_nonlinear_inversion/TiltCopter/To body from Earth ==
  data: Alpha_e input; Earth input; body output
 function body = Tbe(Alpha_e, Earth)
%#codegen
phi = Alpha_e(1);
theta = Alpha_e(2);
psi = Alpha_e(3);

Sphi = sin(phi);
Cphi = cos(phi);
Stheta = sin(theta);
Ctheta = cos(theta);
Spsi = sin(psi);
Cpsi = cos(psi);

TBE = [        Ctheta*Cpsi               Ctheta*Spsi          -Stheta    ;
       Sphi*Stheta*Cpsi-Cphi*Spsi Sphi*Stheta*Spsi+Cphi*Cpsi Sphi*Ctheta ;
       Cphi*Stheta*Cpsi+Sphi*Spsi Cphi*Stheta*Spsi-Sphi*Cpsi Cphi*Ctheta];

body = TBE* Earth;

== matlab function Simulator_nonlinear_inversion/TiltCopter/To Earth from body ==
  data: Alpha_e input; Earth output; body input
 function Earth = Tbet(Alpha_e, body)
%#codegen
phi = Alpha_e(1);
theta = Alpha_e(2);
psi = Alpha_e(3);

Sphi = sin(phi);
Cphi = cos(phi);
Stheta = sin(theta);
Ctheta = cos(theta);
Spsi = sin(psi);
Cpsi = cos(psi);

TBE = [        Ctheta*Cpsi               Ctheta*Spsi          -Stheta    ;
       Sphi*Stheta*Cpsi-Cphi*Spsi Sphi*Stheta*Spsi+Cphi*Cpsi Sphi*Ctheta ;
       Cphi*Stheta*Cpsi+Sphi*Spsi Cphi*Stheta*Spsi-Sphi*Cpsi Cphi*Ctheta];
TEB = TBE';

Earth = TEB* body;

== matlab function Simulator_nonlinear_inversion/TiltCopter/To Earth from body_rates ==
  data: Alpha_e input; Rates_B input; Rates_E output
 function Rates_E = Einv(Alpha_e, Rates_B)
%#codegen
phi = Alpha_e(1);
theta = Alpha_e(2);

Sphi = sin(phi);
Cphi = cos(phi);
Ctheta = cos(theta);
Ttheta = tan(theta);

Einv = [1   Sphi*Ttheta    Cphi*Ttheta ;
        0       Cphi          -Sphi    ;
        0   Sphi/Ctheta    Cphi/Ctheta];

Rates_E = Einv* Rates_B;

== matlab function Simulator_nonlinear_inversion/TiltCopter/Actuators/Traslational Force_1/R_BP1 ==
  data: Rotation_matrix output; alpha_1 input
function Rotation_matrix = fcn(alpha_1)
%#codegen

% Rotation matrix from group propeller 1 to body
R_BP1 = [ 1,0,0; 0, cos(alpha_1), -sin(alpha_1);0, sin(alpha_1),cos(alpha_1)];
      



Rotation_matrix = R_BP1;
